simulink model "pigeon_rb300_task"  (Simulink 3.00)
libraries: genlib x3, mathlib x3, arclib x1

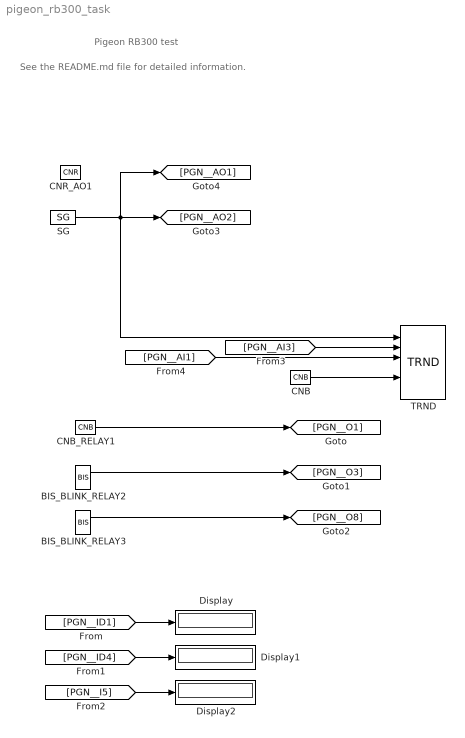
== system pigeon_rb300_task ==
  note: See the README.md file for detailed information.
  note: Pigeon RB300 test
  BIS_BLINK_RELAY2 : genlib/BIS  Y0=Off  t1=1  t2=2  t3=0  t4=4  t5=5  t6=6  t7=7  t8=8  RPT=on  bEdit=off
  BIS_BLINK_RELAY3 : genlib/BIS  Y0=Off  t1=0  t2=0.2  t3=0.4  t4=0.6  t5=0.8  t6=1.0  t7=2.0  t8=0  RPT=on  bEdit=off
  CNB : mathlib/CNB  YCN=on
  CNB_RELAY1 : mathlib/CNB  YCN=on
  CNR_AO1 : mathlib/CNR  ycn=7.5
  Display : Display
      settings: Format=Best fit
  Display1 : Display
      settings: Format=Best fit
  Display2 : Display
      settings: Format=Best fit
  SG : genlib/SG  isig=1: SINE  amp=5  freq=1  phase=0  offset=5  ifrunit=1: Hz  iphunit=1: degrees
  TRND : arclib/TRND  n=4  l=1000  btype=8: Double  ptype1=1: Store  ptype2=1: Store  ptype3=1: Store  ptype4=1: Store  pfac=1  afac=0  arc=0  id=1  Title=Trend Title  timesrc=1: CORETIMER
  wires:
  BIS_BLINK_RELAY2/1 -> [PGN__O3]
  BIS_BLINK_RELAY3/1 -> [PGN__O8]
  CNB/1 -> TRND/5
  CNB_RELAY1/1 -> [PGN__O1]
  [PGN__ID1] -> Display/1
  [PGN__ID4] -> Display1/1
  [PGN__I5] -> Display2/1
  [PGN__AI3] -> TRND/2
  [PGN__AI1] -> TRND/3
  SG/1 -> [PGN__AO2], [PGN__AO1], TRND/1
